simulink model "ClosedLoop_sim"  (R2018b)
settings: Solver=VariableStepAuto  StartTime=0.0  StopTime=10.0  RelTol=1e-3
settings Model: Creator=manzand  LastModifiedBy=manzand

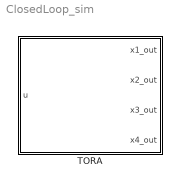
== system ClosedLoop_sim ==
  TORA : Stateflow chart  TreatAsAtomicUnit=on

== stateflow chart ClosedLoop_sim/TORA ==
  settings: updateMethod=CONTINUOUS
  state TORA
    du:
    x1_dot = x2;
    x2_dot = -x1 + 0.1*sin(x3);
    x3_dot = x(4);
    x4_dor = u;
    %OUTPUTS
    x1_out = x1;
    x2_out = x2;
    x3_out = x3;
    x4_out = x4;
  (default) -> TORA : {x1 = 0.65;
      | x2 = -0.65;
      | x3 = -0.35;
      | x4 = 0.55;}
  data: u input; x1_out output; x2_out output; x3_out output; x4_out output; x1 local; x2 local; x3 local; x4 local
  data x1 settings: updateMethod=SF_CONTINUOUS_TIME_DATA
  data x2 settings: updateMethod=SF_CONTINUOUS_TIME_DATA
  data x3 settings: updateMethod=SF_CONTINUOUS_TIME_DATA
  data x4 settings: updateMethod=SF_CONTINUOUS_TIME_DATA
